simulink model "stateflow_image"  (R2015b)
settings: Solver=VariableStepAuto  StartTime=0.0  StopTime=10.0  RelTol=1e-3
settings Model: Creator=ladmin  LastModifiedBy=ladmin

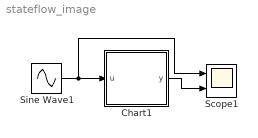
== system stateflow_image ==
  Chart1 : Stateflow chart  TreatAsAtomicUnit=on
  Scope1 : Scope  NumInputPorts=2
  Sine Wave1 : Sin  SampleTime=0
  wires:
  Chart1/1(y) -> Scope1/2
  Sine Wave1/1 -> Scope1/1, Chart1/1(u)

== stateflow chart stateflow_image/Chart1 ==
  note: flip vertical
  note: ?
  note: ?
  note: ?
  note: ?
  note: flip horizontal
  note: rotate 180°
  data: u input; y output
